simulink model "stabilitate"  (R2024a)
settings: Solver=VariableStepAuto  StartTime=0.0  StopTime=10  RelTol=1e-3
values from neighbouring files (symbols this model uses):
  k = 1.5    [parametrii.m]
settings Model: Creator=paulhondola  LastModifiedBy=paulhondola

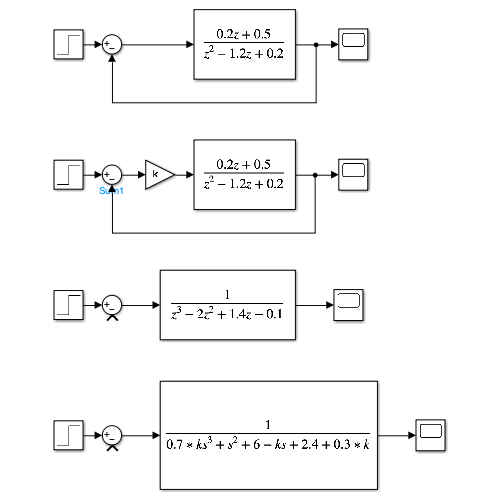
[thumbnail: Simulink's stored preview of the top-level diagram]
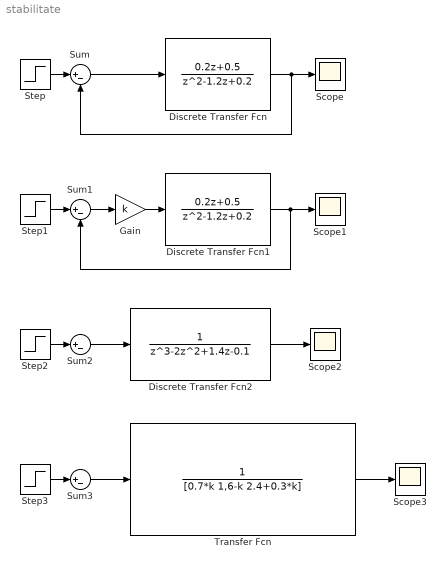
== system stabilitate ==
  Discrete Transfer Fcn : DiscreteTransferFcn  Numerator=[0.2 0.5]  Denominator=[1 -1.2 0.2]  SampleTime=0.05
  Discrete Transfer Fcn1 : DiscreteTransferFcn  Numerator=[0.2 0.5]  Denominator=[1 -1.2 0.2]  SampleTime=0.02
  Discrete Transfer Fcn2 : DiscreteTransferFcn  Denominator=[1 -2 1.4 -0.1]  SampleTime=0.1
  Gain : Gain  Gain=k
  Scope{,1..3} (4 alike) : Scope
  Step{,1..3} (4 alike) : Step  After=5  SampleTime=0
  Sum{,1..3} (4 alike) : Sum  Inputs=|+-
  Transfer Fcn : TransferFcn  Denominator=[0.7*k 1,6-k 2.4+0.3*k]
  wires:
  Gain/1 -> Discrete Transfer Fcn1/1
  Step/1 -> Sum/1
  Step1/1 -> Sum1/1
  Sum1/1 -> Gain/1
  Discrete Transfer Fcn2/1 -> Scope2/1
  Discrete Transfer Fcn1/1 -> Sum1/2, Scope1/1
  Discrete Transfer Fcn/1 -> Sum/2, Scope/1
  Sum/1 -> Discrete Transfer Fcn/1
  Sum2/1 -> Discrete Transfer Fcn2/1
  Step2/1 -> Sum2/1
  Step3/1 -> Sum3/1
  Transfer Fcn/1 -> Scope3/1
  Sum3/1 -> Transfer Fcn/1
